simulink library "INT_EGRVlv_VDSens"  (R2016b)
settings: Solver=VariableStepAuto  StartTime=0.0  StopTime=10.0  RelTol=1e-3
settings Model: Creator=zhulinfeng  LastModifiedBy=zhulinfeng

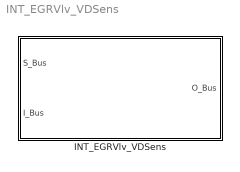
== system INT_EGRVlv_VDSens ==
  INT_EGRVlv_VDSens : Subsystem

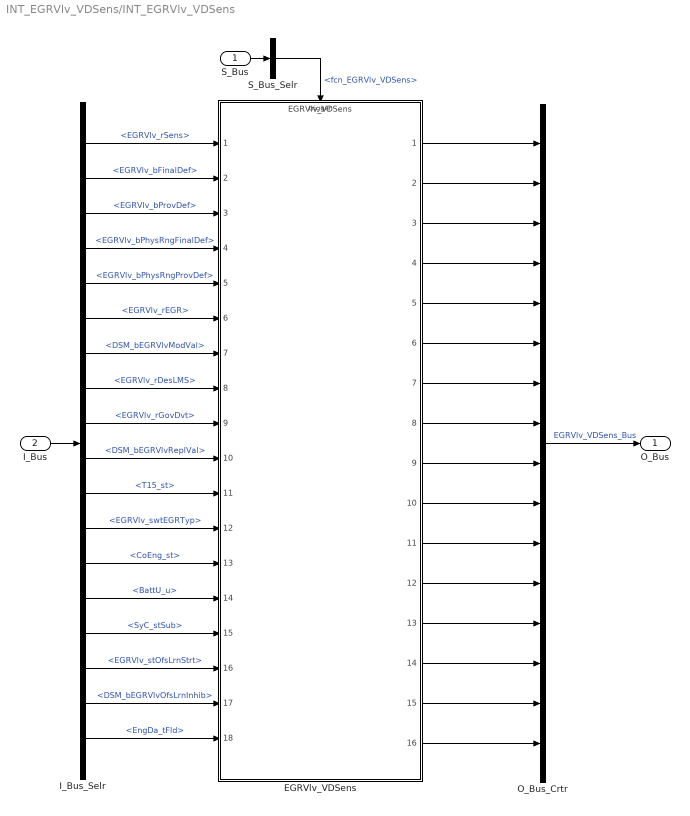
== system INT_EGRVlv_VDSens/INT_EGRVlv_VDSens ==
  S_Bus : Inport
  I_Bus : Inport  Port=2
  EGRVlv_VDSens : ModelReference  ModelNameDialog=EGRVlv_VDSens  SimulationMode=Normal  ModelReferenceVersion=1.53  TriggerPortName=function  TriggerPortTriggerType=function-call  TriggerPortStatesWhenEnabling=held
  I_Bus_Selr : BusSelector  OutputSignals=EGRVlv_rSens,EGRVlv_bFinalDef,EGRVlv_bProvDef,EGRVlv_bPhysRngFinalDef,EGRVlv_bPhysRngProvDef,EGRVlv_rEGR,DSM_bEGRVlvModVal,EGRVlv_rDesLMS,EGRVlv_rGovDvt,DSM_bEGRVlvReplVal,T15_st,EGRVlv_swtEGRTyp,CoEng_st,BattU_u,SyC_stSub,EGRVlv_stOfsLrnStrt,DSM_bEGRVlvOfsLrnInhib,EngDa_tFld
  O_Bus_Crtr : BusCreator  Inputs=16
  S_Bus_Selr : BusSelector  OutputSignals=fcn_EGRVlv_VDSens
  O_Bus : Outport
  wires:
  S_Bus_Selr/1 -> EGRVlv_VDSens/Trigger  "<fcn_EGRVlv_VDSens>"
  S_Bus/1 -> S_Bus_Selr/1
  I_Bus/1 -> I_Bus_Selr/1
  I_Bus_Selr/1 -> EGRVlv_VDSens/1  "<EGRVlv_rSens>"
  I_Bus_Selr/2 -> EGRVlv_VDSens/2  "<EGRVlv_bFinalDef>"
  I_Bus_Selr/3 -> EGRVlv_VDSens/3  "<EGRVlv_bProvDef>"
  I_Bus_Selr/4 -> EGRVlv_VDSens/4  "<EGRVlv_bPhysRngFinalDef>"
  I_Bus_Selr/5 -> EGRVlv_VDSens/5  "<EGRVlv_bPhysRngProvDef>"
  I_Bus_Selr/6 -> EGRVlv_VDSens/6  "<EGRVlv_rEGR>"
  I_Bus_Selr/7 -> EGRVlv_VDSens/7  "<DSM_bEGRVlvModVal>"
  I_Bus_Selr/8 -> EGRVlv_VDSens/8  "<EGRVlv_rDesLMS>"
  I_Bus_Selr/9 -> EGRVlv_VDSens/9  "<EGRVlv_rGovDvt>"
  I_Bus_Selr/10 -> EGRVlv_VDSens/10  "<DSM_bEGRVlvReplVal>"
  I_Bus_Selr/11 -> EGRVlv_VDSens/11  "<T15_st>"
  I_Bus_Selr/12 -> EGRVlv_VDSens/12  "<EGRVlv_swtEGRTyp>"
  I_Bus_Selr/13 -> EGRVlv_VDSens/13  "<CoEng_st>"
  I_Bus_Selr/14 -> EGRVlv_VDSens/14  "<BattU_u>"
  I_Bus_Selr/15 -> EGRVlv_VDSens/15  "<SyC_stSub>"
  I_Bus_Selr/16 -> EGRVlv_VDSens/16  "<EGRVlv_stOfsLrnStrt>"
  I_Bus_Selr/17 -> EGRVlv_VDSens/17  "<DSM_bEGRVlvOfsLrnInhib>"
  I_Bus_Selr/18 -> EGRVlv_VDSens/18  "<EngDa_tFld>"
  O_Bus_Crtr/1 -> O_Bus/1  "EGRVlv_VDSens_Bus"
  EGRVlv_VDSens/1 -> O_Bus_Crtr/1
  EGRVlv_VDSens/2 -> O_Bus_Crtr/2
  EGRVlv_VDSens/3 -> O_Bus_Crtr/3
  EGRVlv_VDSens/4 -> O_Bus_Crtr/4
  EGRVlv_VDSens/5 -> O_Bus_Crtr/5
  EGRVlv_VDSens/6 -> O_Bus_Crtr/6
  EGRVlv_VDSens/7 -> O_Bus_Crtr/7
  EGRVlv_VDSens/8 -> O_Bus_Crtr/8
  EGRVlv_VDSens/9 -> O_Bus_Crtr/9
  EGRVlv_VDSens/10 -> O_Bus_Crtr/10
  EGRVlv_VDSens/11 -> O_Bus_Crtr/11
  EGRVlv_VDSens/12 -> O_Bus_Crtr/12
  EGRVlv_VDSens/13 -> O_Bus_Crtr/13
  EGRVlv_VDSens/14 -> O_Bus_Crtr/14
  EGRVlv_VDSens/15 -> O_Bus_Crtr/15
  EGRVlv_VDSens/16 -> O_Bus_Crtr/16
